simulink model "ex_01_model"  (R2014a)
settings: Solver=ode45  StartTime=0.0  StopTime=10  RelTol=1e-3
undefined symbols (not defined in the file): G, x, y, z
settings Model: Creator=Nino  LastModifiedBy=Nino

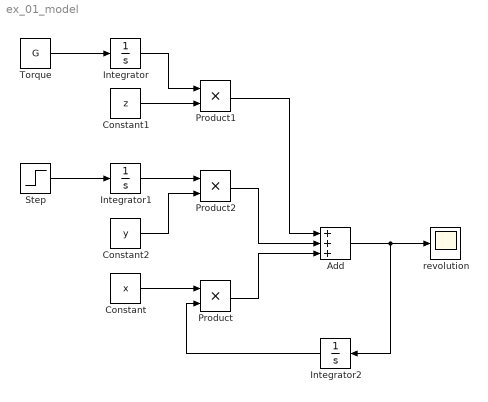
== system ex_01_model ==
  Add : Sum  Inputs=+++
  Constant : Constant  Value=x
  Constant1 : Constant  Value=z
  Constant2 : Constant  Value=y
  Integrator : Integrator
  Integrator1 : Integrator
  Integrator2 : Integrator
  Product : Product
  Product1 : Product
  Product2 : Product
  Step : Step  After=5  SampleTime=0
  Torque : Constant  Value=G
  revolution : Scope
  wires:
  Integrator2/1 -> Product/2
  Constant/1 -> Product/1
  Product/1 -> Add/3
  Add/1 -> Integrator2/1, revolution/1
  Integrator1/1 -> Product2/1
  Constant2/1 -> Product2/2
  Product2/1 -> Add/2
  Constant1/1 -> Product1/2
  Integrator/1 -> Product1/1
  Product1/1 -> Add/1
  Torque/1 -> Integrator/1
  Step/1 -> Integrator1/1
